simulink model "Vicon_Raw_Data_Collection"  (R2012b)
settings: Solver=ode5  StartTime=0.0  StopTime=inf  FixedStep=sample_time  RelTol=1e-3
InitFcn:
  | sample_time=0.005;%0.004;%0.0025;%0.02;
  | sample_time_Vicon = 0.005;
  | DeltaT = 0.02;
  | g = 9.81;
  | H0 = g%0.3165;
  | Kl = 1;
  | 
  | Q6_mass = 0.8;
  | 
  | Q6_Omega_r = 1.2; %for horizon ref
  | Q6_Zeta_r = 0.707; %for horizon ref
  | Q6_Omega_r_h = 2;%for vertical ref
  | Q6_Zeta_r_h = 0.7; %for vertical ref
  | 
  | 
  | Q6_Omega = 1.5; %for horizon control
  | Q6_Zeta = 0.507; %for horizon control
  | Q6_Omega_h= 2 %for vertical control
  | Q6_Zeta_h = 0.5; %for vertical control
  | 
  | 
  | Q6_acc_max = 5;%horizontal max acc
  | Q6_acc_max_h = 5;%horizontal max acc
  | 
  | omega_circle = 10*pi/180;
  | 
  | omega_h = 0.1;%Ascending speed
  | PI = pi;
  | Circle_R = 2;
  | 
  | 
  | MAX_Height = -2;
  | 
  | 
  | % for NN
  | n = 5;
  | r = 3;
  | n2 = 5;
  | NN_ST = 0.02;
  | 
  | GAMA_V = 6;
  | gama_V_e = 0.01;
  | 
  | GAMA_W = GAMA_V;
  | gama_W_e =0.01;
  | 
  | % deadzone
  | NN_Deadzone_Z = 0;
  | 
  | % inputs nomalizaton parameters
  | NN_Z_y_min = -3;
  | NN_Z_y_max = 0.5;
  | 
  | NN_Z_v_max = 8;
  | NN_Z_v_min = -NN_Z_v_max;
  | 
  | % alpha = 0.034;
  | alpha = 1;
  | % c_f = 0.0015;
  | c_f = 0.001;
  | c_y_tilt = 1*0.5;
libraries: simulink x2
settings Model: Creator=ttcl3  LastModifiedBy=airshow
settings SolverCC: MaxConsecutiveMinStep=auto
settings DataIOCC: SignalLoggingSaveFormat=ModelDataLogs
settings DebuggingCC: MultiTaskRateTransMsg=warning  FcnCallInpInsideContextMsg=UseLocalSettings
settings SFSimCC: SimParseCustomCode=off
settings GRTTargetCC: CombineOutputUpdateFcns=off  GRTInterface=on

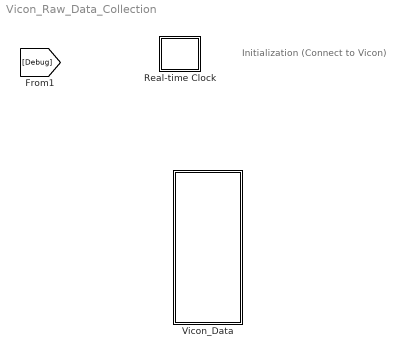
== system Vicon_Raw_Data_Collection ==
  note: Initialization
      | (Connect to Vicon)
  Real-time Clock : Subsystem  mask(Real-time Clock){sample_time=0.02, tolerance=1}
      mask prompts: sample_time "Synchronize with real-time every n seconds:"; tolerance "Real-time warning tolerance (seconds):"
      mask help: Real-time Synchronization Block
      mask Help: This block synchronizes simulation time with the PC real-time clock or UNIX system clock. The first dialog entry is the period at which the clock is checked to insure real-time synchronization. The second dialog entry is the number of seconds that the simulation time must be within real-time before a warning is printed.
      mask Display: plot(0,0,100,100,[40,60,60,54,54,64,69,76,82,77,81,83,83,81,78,74,70,64,57,49,41,35,32,30,30,31,34,40,47,47,40,40],[90,90,85,85,80,79,76,87,80,70,64,57,49,41,33,28,24,22,21,23,25,31,37,46,56,65,73,78,80,85,85,90],[69,53,53],[64,50,73])
  Vicon_Data : Subsystem

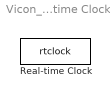
== system Vicon_Raw_Data_Collection/Real-time Clock ==
  Real-time Clock : S-Function  FunctionName=rtclock  Parameters=sample_time, tolerance  EnableBusSupport=off

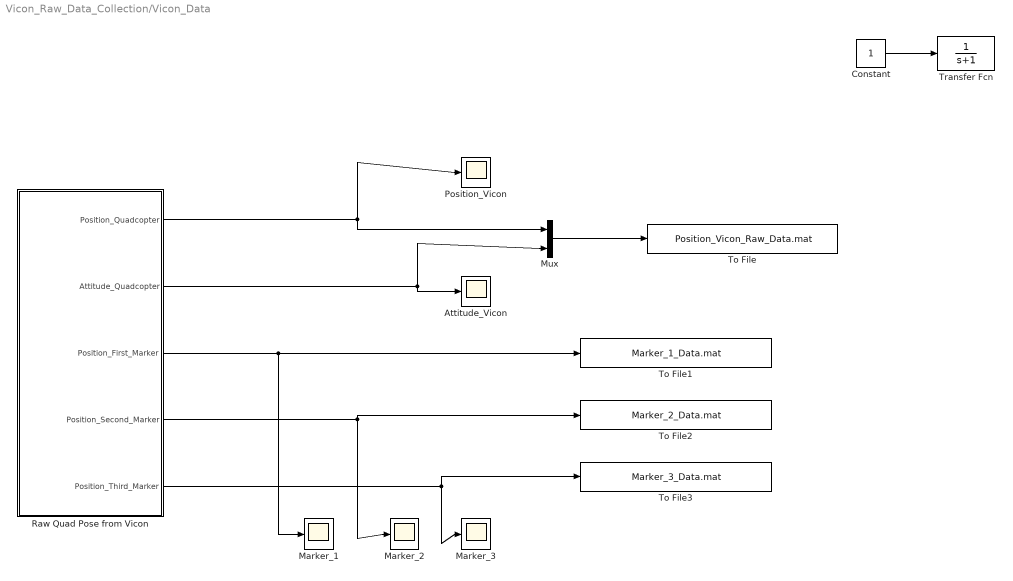
== system Vicon_Raw_Data_Collection/Vicon_Data ==
  Attitude_Vicon : Scope
      settings: YMin=0  YMax=3.25
  Constant : Constant  SampleTime=5
  Marker_1 : Scope
      settings: YMin=0  YMax=3.25  SaveName=ScopeData2
  Marker_2 : Scope
      settings: YMin=0  YMax=3.25  SaveName=ScopeData3
  Marker_3 : Scope
      settings: YMin=0  YMax=3.25  SaveName=ScopeData4
  Mux : Mux  Inputs=2
  Position_Vicon : Scope
      settings: YMin=-0.25  YMax=3
  Raw Quad Pose from Vicon : Subsystem
  To File : ToFile  Filename=Position_Vicon_Raw_Data.mat  SaveFormat=Timeseries
  To File1 : ToFile  Filename=Marker_1_Data.mat  SaveFormat=Timeseries
  To File2 : ToFile  Filename=Marker_2_Data.mat  SaveFormat=Timeseries
  To File3 : ToFile  Filename=Marker_3_Data.mat  SaveFormat=Timeseries
  Transfer Fcn : TransferFcn  Denominator=[1 1]
  wires:
  Constant/1 -> Transfer Fcn/1
  Raw Quad Pose from Vicon/1(Position_Quadcopter) -> Position_Vicon/1, Mux/1
  Raw Quad Pose from Vicon/2(Attitude_Quadcopter) -> Mux/2, Attitude_Vicon/1
  Mux/1 -> To File/1
  Raw Quad Pose from Vicon/3(Position_First_Marker) -> Marker_1/1, To File1/1
  Raw Quad Pose from Vicon/4(Position_Second_Marker) -> Marker_2/1, To File2/1
  Raw Quad Pose from Vicon/5(Position_Third_Marker) -> Marker_3/1, To File3/1

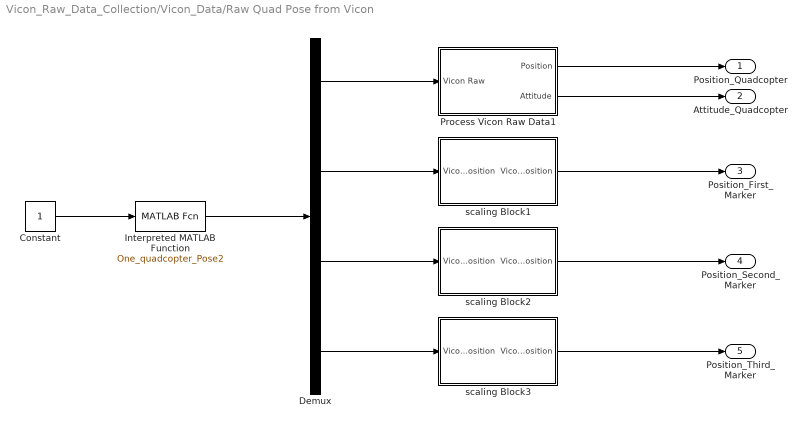
== system Vicon_Raw_Data_Collection/Vicon_Data/Raw Quad Pose from Vicon ==
  Constant : Constant  SampleTime=sample_time
  Demux : Demux
  Interpreted MATLAB Function : MATLABFcn  MATLABFcn=One_quadcopter_Pose2
  Process Vicon Raw Data1 : Subsystem
  scaling Block1 : Subsystem
  scaling Block2 : Subsystem
  scaling Block3 : Subsystem
  Position_Quadcopter : Outport
  Attitude_Quadcopter : Outport  Port=2
  Position_First_Marker : Outport  Port=3
  Position_Second_Marker : Outport  Port=4
  Position_Third_Marker : Outport  Port=5
  wires:
  Interpreted MATLAB Function/1 -> Demux/1
  Constant/1 -> Interpreted MATLAB Function/1
  Process Vicon Raw Data1/2(Attitude) -> Attitude_Quadcopter/1
  Process Vicon Raw Data1/1(Position) -> Position_Quadcopter/1
  Demux/1 -> Process Vicon Raw Data1/1(Vicon Raw)
  Demux/2 -> scaling Block1/1(Vicon Raw Position)
  Demux/3 -> scaling Block2/1(Vicon Raw Position)
  Demux/4 -> scaling Block3/1(Vicon Raw Position)
  scaling Block1/1(Vicon Position) -> Position_First_Marker/1
  scaling Block2/1(Vicon Position) -> Position_Second_Marker/1
  scaling Block3/1(Vicon Position) -> Position_Third_Marker/1

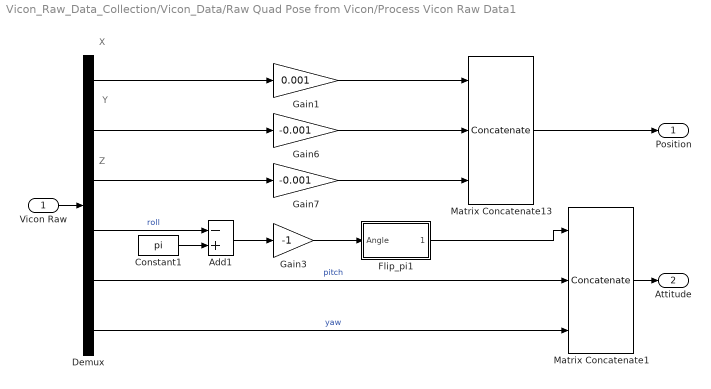
== system Vicon_Raw_Data_Collection/Vicon_Data/Raw Quad Pose from Vicon/Process Vicon Raw Data1 ==
  note: X
  note: Y
  note: Z
  Vicon Raw : Inport
  Add1 : Sum  Inputs=-+
  Constant1 : Constant  Value=pi  OutDataTypeStr=double
  Demux : Demux  Outputs=6
  Flip_pi1 : Subsystem  mask(Flip -pi to pi){}
      mask help: Flips the inputs into the range -pi to pi
      mask Help: Flips the inputs into the range -pi to pi
      mask Display: disp('Flip_pi')
  Gain1 : Gain  Gain=0.001
  Gain3 : Gain  Gain=-1
  Gain6 : Gain  Gain=-0.001
  Gain7 : Gain  Gain=-0.001
  Matrix Concatenate1 : Concatenate  NumInputs=3  Mode=Multidimensional array
  Matrix Concatenate13 : Concatenate  NumInputs=3  Mode=Multidimensional array
  Position : Outport
  Attitude : Outport  Port=2
  wires:
  Constant1/1 -> Add1/2
  Demux/6 -> Matrix Concatenate1/3  "yaw"
  Gain1/1 -> Matrix Concatenate13/1
  Demux/1 -> Gain1/1
  Demux/2 -> Gain6/1
  Demux/3 -> Gain7/1
  Demux/4 -> Add1/1  "roll"
  Gain6/1 -> Matrix Concatenate13/2
  Gain7/1 -> Matrix Concatenate13/3
  Add1/1 -> Gain3/1
  Gain3/1 -> Flip_pi1/1(Angle)
  Demux/5 -> Matrix Concatenate1/2  "pitch"
  Flip_pi1/1(Angle_Flip) -> Matrix Concatenate1/1
  Matrix Concatenate13/1 -> Position/1
  Vicon Raw/1 -> Demux/1
  Matrix Concatenate1/1 -> Attitude/1

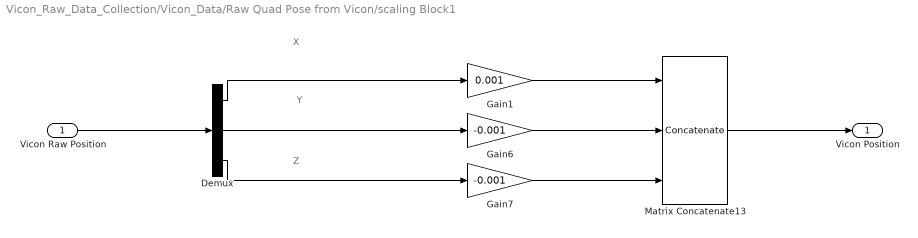
== system Vicon_Raw_Data_Collection/Vicon_Data/Raw Quad Pose from Vicon/scaling Block1 ==
  note: Z
  note: Y
  note: X
  Vicon Raw Position : Inport
  Demux : Demux  Outputs=3
  Gain1 : Gain  Gain=0.001
  Gain6 : Gain  Gain=-0.001
  Gain7 : Gain  Gain=-0.001
  Matrix Concatenate13 : Concatenate  NumInputs=3  Mode=Multidimensional array
  Vicon Position : Outport
  wires:
  Vicon Raw Position/1 -> Demux/1
  Matrix Concatenate13/1 -> Vicon Position/1
  Gain7/1 -> Matrix Concatenate13/3
  Gain6/1 -> Matrix Concatenate13/2
  Demux/3 -> Gain7/1
  Demux/2 -> Gain6/1
  Demux/1 -> Gain1/1
  Gain1/1 -> Matrix Concatenate13/1

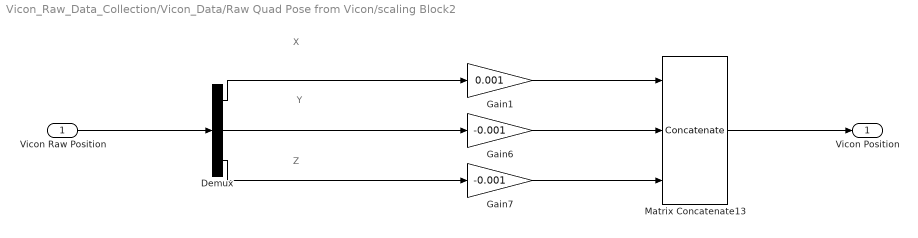
== system Vicon_Raw_Data_Collection/Vicon_Data/Raw Quad Pose from Vicon/scaling Block2 ==
  note: X
  note: Y
  note: Z
  Vicon Raw Position : Inport
  Demux : Demux  Outputs=3
  Gain1 : Gain  Gain=0.001
  Gain6 : Gain  Gain=-0.001
  Gain7 : Gain  Gain=-0.001
  Matrix Concatenate13 : Concatenate  NumInputs=3  Mode=Multidimensional array
  Vicon Position : Outport
  wires:
  Gain1/1 -> Matrix Concatenate13/1
  Demux/1 -> Gain1/1
  Demux/2 -> Gain6/1
  Demux/3 -> Gain7/1
  Gain6/1 -> Matrix Concatenate13/2
  Gain7/1 -> Matrix Concatenate13/3
  Matrix Concatenate13/1 -> Vicon Position/1
  Vicon Raw Position/1 -> Demux/1

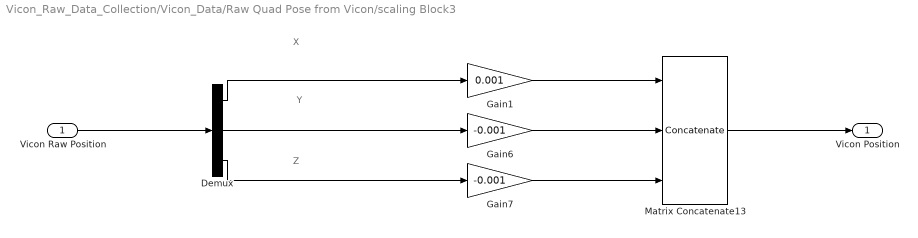
== system Vicon_Raw_Data_Collection/Vicon_Data/Raw Quad Pose from Vicon/scaling Block3 ==
  note: Z
  note: Y
  note: X
  Vicon Raw Position : Inport
  Demux : Demux  Outputs=3
  Gain1 : Gain  Gain=0.001
  Gain6 : Gain  Gain=-0.001
  Gain7 : Gain  Gain=-0.001
  Matrix Concatenate13 : Concatenate  NumInputs=3  Mode=Multidimensional array
  Vicon Position : Outport
  wires:
  Vicon Raw Position/1 -> Demux/1
  Matrix Concatenate13/1 -> Vicon Position/1
  Gain7/1 -> Matrix Concatenate13/3
  Gain6/1 -> Matrix Concatenate13/2
  Demux/3 -> Gain7/1
  Demux/2 -> Gain6/1
  Demux/1 -> Gain1/1
  Gain1/1 -> Matrix Concatenate13/1

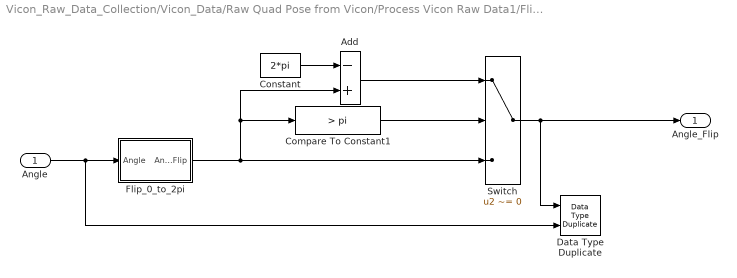
== system Vicon_Raw_Data_Collection/Vicon_Data/Raw Quad Pose from Vicon/Process Vicon Raw Data1/Flip_pi1 ==
  Angle : Inport
  Add : Sum  Inputs=-+
  Compare To Constant1 : simulink/Logic and Bit Operations/Compare To Constant  relop=>  const=pi  OutDataTypeStr=uint8  ZeroCross=off
  Constant : Constant  Value=2*pi
  Data Type Duplicate : DataTypeDuplicate
  Flip_0_to_2pi : Subsystem  mask(Flip zero to 2pi){}
      mask help: Flips the inputs into the range zero to +2pi
      mask Help: Flips the inputs into the range zero to +2pi
      mask Display: disp('Flip_0_2pi')
  Switch : Switch  Criteria=u2 ~= 0
  Angle_Flip : Outport
  wires:
  Switch/1 -> Data Type Duplicate/1, Angle_Flip/1
  Add/1 -> Switch/1
  Constant/1 -> Add/1
  Compare To Constant1/1 -> Switch/2
  Flip_0_to_2pi/1(Angle_Flip) -> Add/2, Compare To Constant1/1, Switch/3
  Angle/1 -> Data Type Duplicate/2, Flip_0_to_2pi/1(Angle)

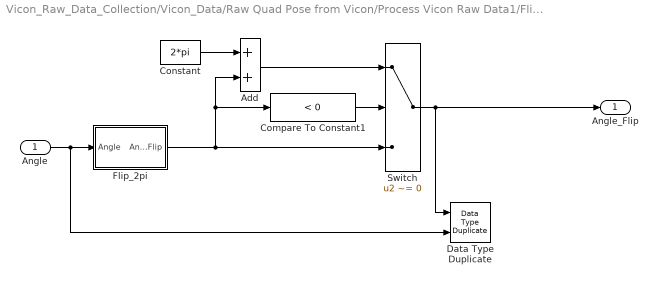
== system Vicon_Raw_Data_Collection/Vicon_Data/Raw Quad Pose from Vicon/Process Vicon Raw Data1/Flip_pi1/Flip_0_to_2pi ==
  Angle : Inport
  Add : Sum
  Compare To Constant1 : simulink/Logic and Bit Operations/Compare To Constant  relop=<  const=0  OutDataTypeStr=uint8  ZeroCross=off
  Constant : Constant  Value=2*pi
  Data Type Duplicate : DataTypeDuplicate
  Flip_2pi : Subsystem  mask(Flip -2pi to 2pi){}
      mask help: Flips the inputs into the range -2pi to +2pi
      mask Help: Flips the inputs into the range -2pi to +2pi
      mask Display: disp('Flip_2pi')
  Switch : Switch  Criteria=u2 ~= 0
  Angle_Flip : Outport
  wires:
  Switch/1 -> Data Type Duplicate/1, Angle_Flip/1
  Angle/1 -> Data Type Duplicate/2, Flip_2pi/1(Angle)
  Add/1 -> Switch/1
  Constant/1 -> Add/1
  Compare To Constant1/1 -> Switch/2
  Flip_2pi/1(Angle_Flip) -> Switch/3, Add/2, Compare To Constant1/1

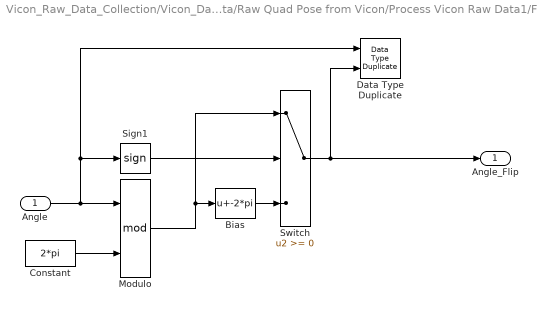
== system Vicon_Raw_Data_Collection/Vicon_Data/Raw Quad Pose from Vicon/Process Vicon Raw Data1/Flip_pi1/Flip_0_to_2pi/Flip_2pi ==
  Angle : Inport
  Bias : Bias  Bias=-2*pi
  Constant : Constant  Value=2*pi
  Data Type Duplicate : DataTypeDuplicate
  Modulo : Math  Operator=mod  SaturateOnIntegerOverflow=on
  Sign1 : Signum
  Switch : Switch
  Angle_Flip : Outport
  wires:
  Switch/1 -> Data Type Duplicate/2, Angle_Flip/1
  Bias/1 -> Switch/3
  Sign1/1 -> Switch/2
  Modulo/1 -> Switch/1, Bias/1
  Constant/1 -> Modulo/2
  Angle/1 -> Data Type Duplicate/1, Sign1/1, Modulo/1
